simulink model "Clth"  (R2016b)
settings: Solver=VariableStepAuto  StartTime=0.0  StopTime=10.0  RelTol=1e-3
settings Model: Creator=jiakui  LastModifiedBy=jiakui

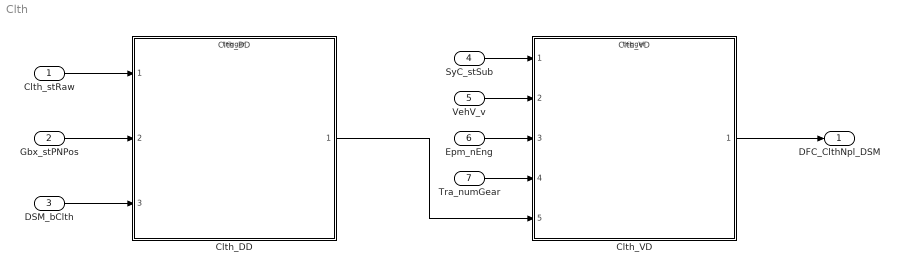
== system Clth ==
  Clth_stRaw : Inport  Description=Raw signal of clutch state  OutMin=0  OutMax=255  OutDataTypeStr=State_uint8
  Gbx_stPNPos : Inport  Description=Park Neutral Switch status  Port=2  OutMin=0  OutMax=255  OutDataTypeStr=State_uint8
  DSM_bClth : Inport  Description=state of Fid_Clth  Port=3  OutMin=0  OutMax=1  OutDataTypeStr=boolean
  SyC_stSub : Inport  Description=Current system/ECU sub-state  Port=4  OutDataTypeStr=Enum: SubSysExeState_conv
  VehV_v : Inport  Tag=km/h  Description=Vehicle speed  Port=5  OutMin=0  OutMax=250  OutDataTypeStr=VehSpeed_km_h
  Epm_nEng : Inport  Tag=rpm  Description=Engine speed  Port=6  OutMin=0  OutMax=6000  OutDataTypeStr=EngSpeed_rpm
  Tra_numGear : Inport  Description=Current gear information  Port=7  OutMin=-128  OutMax=127  OutDataTypeStr=Tra_num
  Clth_DD : ModelReference  ModelNameDialog=Clth_DD  SimulationMode=Normal  ModelReferenceVersion=1.9  TriggerPortName=function  TriggerPortTriggerType=function-call  TriggerPortStatesWhenEnabling=held
  Clth_VD : ModelReference  ModelNameDialog=Clth_VD  SimulationMode=Normal  ModelReferenceVersion=1.10  TriggerPortName=function  TriggerPortTriggerType=function-call  TriggerPortStatesWhenEnabling=held
  DFC_ClthNpl_DSM : Outport  Description="state of error \"DFC_ClthNpl\""  OutMin=0  OutMax=1  OutDataTypeStr=boolean
  wires:
  Gbx_stPNPos/1 -> Clth_DD/2
  Clth_stRaw/1 -> Clth_DD/1
  DSM_bClth/1 -> Clth_DD/3
  Clth_DD/1 -> Clth_VD/5
  VehV_v/1 -> Clth_VD/2
  Epm_nEng/1 -> Clth_VD/3
  Tra_numGear/1 -> Clth_VD/4
  SyC_stSub/1 -> Clth_VD/1
  Clth_VD/1 -> DFC_ClthNpl_DSM/1
